simulink model "FOC_SVPWM_Implementation"  (R2025a)
settings: Solver=FixedStepDiscrete  StartTime=0.0  StopTime=10.0  FixedStep=0.0001  RelTol=1e-3
values from neighbouring files (symbols this model uses):
  dq_decouping_ena = 1.0    [FOV_SVPWM_Algorithm.sldd]
  dq_voltage_ratio = 0.57735026918962584    [FOV_SVPWM_Algorithm.sldd]
  duty_sat_lower = 0.0    [FOV_SVPWM_Algorithm.sldd]
  duty_sat_upper = 100.0    [FOV_SVPWM_Algorithm.sldd]
  I_s_max = 350.0    [FOV_SVPWM_Algorithm.sldd]
  KI_c = 30.0    [FOV_SVPWM_Algorithm.sldd]
  Kp_c = 1.1    [FOV_SVPWM_Algorithm.sldd]
  L_d = 0.0003    [FOV_SVPWM_Algorithm.sldd]
  L_q = 0.0003    [FOV_SVPWM_Algorithm.sldd]
  p = 3.0    [FOV_SVPWM_Algorithm.sldd]
  Psi_p = 0.095    [FOV_SVPWM_Algorithm.sldd]
  svpwm_ena = 1.0    [FOV_SVPWM_Algorithm.sldd]
undefined symbols (not defined in the file or in its folder): DiscIntNeverNeededParam
libraries: simulink x4
settings Model: DataDictionary=FOV_SVPWM_Algorithm.sldd  Creator=RSINGH25  LastModifiedBy=RSINGH25
settings OptimizationCC: DefaultParameterBehavior=Inlined  EnhancedBackFolding=on  PassReuseOutputArgsThreshold=0.0  OptimizeBlockOrder=speed  DifferentSizesBufferReuse=on  OptimizationCustomize=off
settings DebuggingCC: ParameterPrecisionLossMsg=none  ParamSuppressDoubleToSinglePrecisionLossMsg=on  ParameterTunabilityLossMsg=error
settings SFSimCC: MATLABDynamicMemAlloc=off
settings RTWCC: GenCodeOnly=on  GenerateReport=on  LaunchReport=on
settings CodeAppCC: ForceParamTrailComments=on  OperatorAnnotations=on

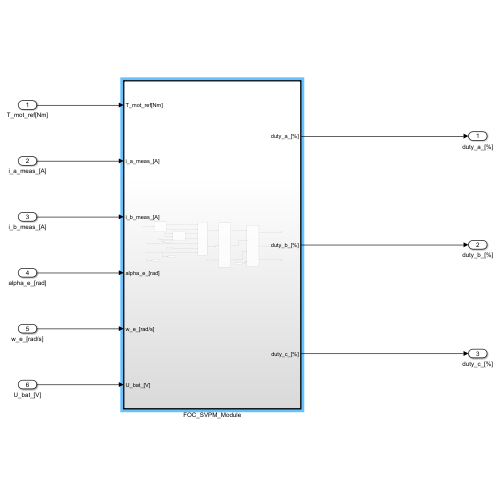
[thumbnail: Simulink's stored preview of the top-level diagram]
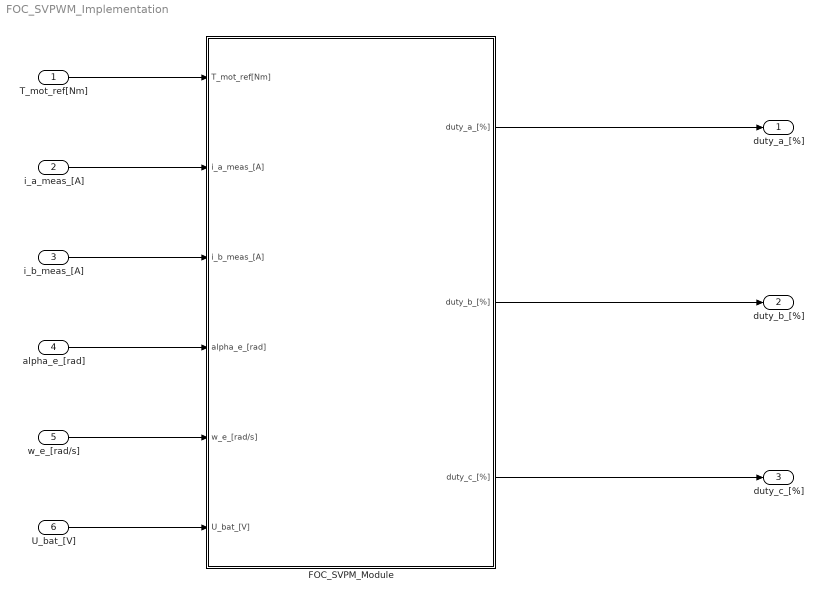
== system FOC_SVPWM_Implementation ==
  T_mot_ref[Nm] : Inport
  i_a_meas_[A] : Inport  Port=2
  i_b_meas_[A] : Inport  Port=3
  alpha_e_[rad] : Inport  Port=4
  w_e_[rad/s] : Inport  Port=5
  U_bat_[V] : Inport  Port=6
  FOC_SVPM_Module : Subsystem  TreatAsAtomicUnit=on
  duty_a_[%] : Outport
  duty_b_[%] : Outport  Port=2
  duty_c_[%] : Outport  Port=3
  wires:
  T_mot_ref[Nm]/1 -> FOC_SVPM_Module/1(T_mot_ref[Nm])
  i_a_meas_[A]/1 -> FOC_SVPM_Module/2(i_a_meas_[A])
  i_b_meas_[A]/1 -> FOC_SVPM_Module/3(i_b_meas_[A])
  alpha_e_[rad]/1 -> FOC_SVPM_Module/4(alpha_e_[rad])
  w_e_[rad/s]/1 -> FOC_SVPM_Module/5(w_e_[rad/s])
  U_bat_[V]/1 -> FOC_SVPM_Module/6(U_bat_[V])
  FOC_SVPM_Module/1(duty_a_[%]) -> duty_a_[%]/1
  FOC_SVPM_Module/2(duty_b_[%]) -> duty_b_[%]/1
  FOC_SVPM_Module/3(duty_c_[%]) -> duty_c_[%]/1

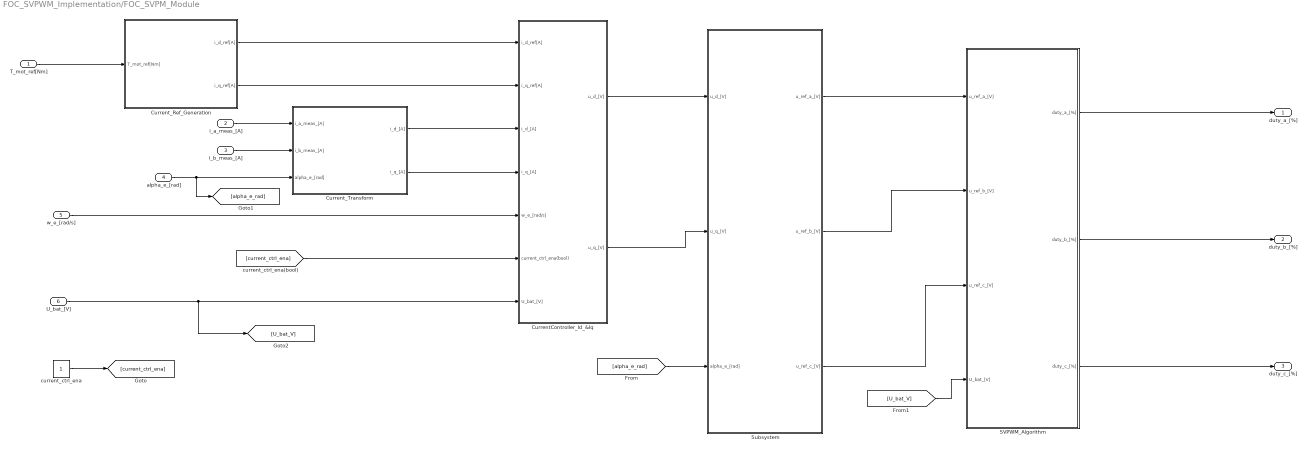
== system FOC_SVPWM_Implementation/FOC_SVPM_Module ==
  T_mot_ref[Nm] : Inport
  i_a_meas_[A] : Inport  Port=2
  i_b_meas_[A] : Inport  Port=3
  alpha_e_[rad] : Inport  Port=4
  w_e_[rad/s] : Inport  Port=5
  U_bat_[V] : Inport  Port=6
  CurrentController_Id_&Iq : Subsystem  TreatAsAtomicUnit=on
  Current_Ref_Generation : Subsystem  TreatAsAtomicUnit=on
  Current_Transform : Subsystem  TreatAsAtomicUnit=on
  SVPWM_Algorithm : Subsystem  TreatAsAtomicUnit=on
  Subsystem : Subsystem  TreatAsAtomicUnit=on
  current_ctrl_ena : Constant
  duty_a_[%] : Outport
  duty_b_[%] : Outport  Port=2
  duty_c_[%] : Outport  Port=3
  wires:
  current_ctrl_ena/1 -> [current_ctrl_ena]
  SVPWM_Algorithm/1(duty_a_[%]) -> duty_a_[%]/1
  Subsystem/2(u_ref_b_[V]) -> SVPWM_Algorithm/2(u_ref_b_[V])
  [current_ctrl_ena] -> CurrentController_Id_&Iq/6(current_ctrl_ena(bool))
  U_bat_[V]/1 -> [U_bat_V], CurrentController_Id_&Iq/7(U_bat_[V])
  Current_Transform/2(i_q_[A]) -> CurrentController_Id_&Iq/4(i_q_[A])
  Subsystem/3(u_ref_c_[V]) -> SVPWM_Algorithm/3(u_ref_c_[V])
  T_mot_ref[Nm]/1 -> Current_Ref_Generation/1(T_mot_ref[Nm])
  alpha_e_[rad]/1 -> [alpha_e_rad], Current_Transform/3(alpha_e_[rad])
  i_a_meas_[A]/1 -> Current_Transform/1(i_a_meas_[A])
  CurrentController_Id_&Iq/2(u_q_[V]) -> Subsystem/2(u_q_[V])
  CurrentController_Id_&Iq/1(u_d_[V]) -> Subsystem/1(u_d_[V])
  Current_Ref_Generation/1(i_d_ref[A]) -> CurrentController_Id_&Iq/1(i_d_ref[A])
  Current_Ref_Generation/2(i_q_ref[A]) -> CurrentController_Id_&Iq/2(i_q_ref[A])
  SVPWM_Algorithm/2(duty_b_[%]) -> duty_b_[%]/1
  Subsystem/1(u_ref_a_[V]) -> SVPWM_Algorithm/1(u_ref_a_[V])
  [U_bat_V] -> SVPWM_Algorithm/4(U_bat_[V])
  Current_Transform/1(i_d_[A]) -> CurrentController_Id_&Iq/3(i_d_[A])
  [alpha_e_rad] -> Subsystem/3(alpha_e_[rad])
  SVPWM_Algorithm/3(duty_c_[%]) -> duty_c_[%]/1
  i_b_meas_[A]/1 -> Current_Transform/2(i_b_meas_[A])
  w_e_[rad/s]/1 -> CurrentController_Id_&Iq/5(w_e_[rad/s])

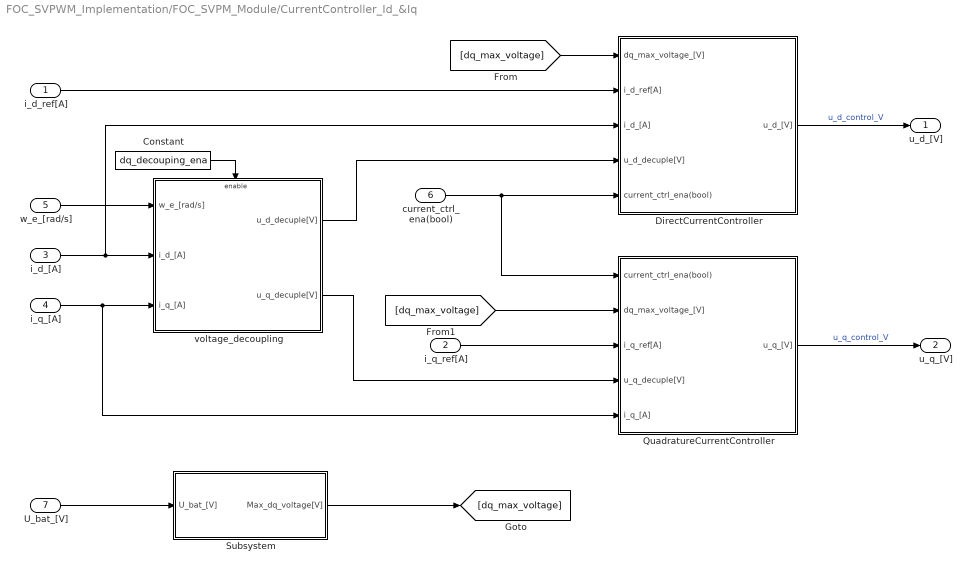
== system FOC_SVPWM_Implementation/FOC_SVPM_Module/CurrentController_Id_&Iq ==
  i_d_ref[A] : Inport
  i_q_ref[A] : Inport  Port=2
  i_d_[A] : Inport  Port=3
  i_q_[A] : Inport  Port=4
  w_e_[rad/s] : Inport  Port=5
  current_ctrl_ena(bool) : Inport  Port=6
  U_bat_[V] : Inport  Port=7
  Constant : Constant  Value=dq_decouping_ena
  DirectCurrentController : Subsystem
  QuadratureCurrentController : Subsystem
  Subsystem : Subsystem
  voltage_decoupling : Subsystem
  u_d_[V] : Outport
  u_q_[V] : Outport  Port=2
  wires:
  w_e_[rad/s]/1 -> voltage_decoupling/1(w_e_[rad/s])
  i_d_[A]/1 -> DirectCurrentController/3(i_d_[A]), voltage_decoupling/2(i_d_[A])
  i_q_[A]/1 -> QuadratureCurrentController/5(i_q_[A]), voltage_decoupling/3(i_q_[A])
  i_d_ref[A]/1 -> DirectCurrentController/2(i_d_ref[A])
  voltage_decoupling/1(u_d_decuple[V]) -> DirectCurrentController/4(u_d_decuple[V])
  current_ctrl_ena(bool)/1 -> QuadratureCurrentController/1(current_ctrl_ena(bool)), DirectCurrentController/5(current_ctrl_ena(bool))
  U_bat_[V]/1 -> Subsystem/1(U_bat_[V])
  Subsystem/1(Max_dq_voltage[V]) -> [dq_max_voltage]
  [dq_max_voltage] -> DirectCurrentController/1(dq_max_voltage_[V])
  i_q_ref[A]/1 -> QuadratureCurrentController/3(i_q_ref[A])
  voltage_decoupling/2(u_q_decuple[V]) -> QuadratureCurrentController/4(u_q_decuple[V])
  [dq_max_voltage] -> QuadratureCurrentController/2(dq_max_voltage_[V])
  DirectCurrentController/1(u_d_[V]) -> u_d_[V]/1  "u_d_control_V"
  QuadratureCurrentController/1(u_q_[V]) -> u_q_[V]/1  "u_q_control_V"
  Constant/1 -> voltage_decoupling/Enable

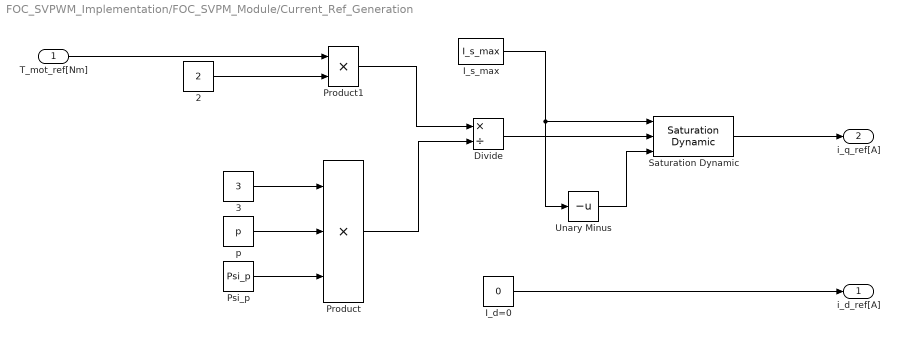
== system FOC_SVPWM_Implementation/FOC_SVPM_Module/Current_Ref_Generation ==
  T_mot_ref[Nm] : Inport
  2 : Constant  Value=2  OutDataTypeStr=single
  3 : Constant  Value=3  OutDataTypeStr=single
  Divide : Product  Inputs=*/
  I_d=0 : Constant  Value=0  OutDataTypeStr=single
  I_s_max : Constant  Value=I_s_max  OutDataTypeStr=single
  Product : Product  Inputs=3
  Product1 : Product
  Psi_p : Constant  Value=Psi_p  OutDataTypeStr=single
  Saturation Dynamic : simulink/Discontinuities/Saturation Dynamic  OutMin=[]  OutMax=[]  OutDataTypeStr=Inherit: Same as second input  OutDataType=fixdt(1, 16)  OutScaling=2^-10  DoSatur=off
  Unary Minus : UnaryMinus
  p : Constant  Value=p  OutDataTypeStr=single
  i_d_ref[A] : Outport
  i_q_ref[A] : Outport  Port=2
  wires:
  3/1 -> Product/1
  Psi_p/1 -> Product/3
  p/1 -> Product/2
  2/1 -> Product1/2
  T_mot_ref[Nm]/1 -> Product1/1
  Product1/1 -> Divide/1
  Product/1 -> Divide/2
  Saturation Dynamic/1 -> i_q_ref[A]/1
  Divide/1 -> Saturation Dynamic/2
  I_s_max/1 -> Unary Minus/1, Saturation Dynamic/1
  Unary Minus/1 -> Saturation Dynamic/3
  I_d=0/1 -> i_d_ref[A]/1

== system FOC_SVPWM_Implementation/FOC_SVPM_Module/Current_Transform ==
  i_a_meas_[A] : Inport
  i_b_meas_[A] : Inport  Port=2
  alpha_e_[rad] : Inport  Port=3
  Clark_transform : Subsystem
  Park_Transform : Subsystem
  i_d_[A] : Outport
  i_q_[A] : Outport  Port=2
  wires:
  i_a_meas_[A]/1 -> Clark_transform/1(i_a_meas_[A])
  i_b_meas_[A]/1 -> Clark_transform/2(i_b_meas_[A])
  Clark_transform/1(i_x_[A]) -> Park_Transform/1(i_x_[A])  "i_x_meas_A"
  Clark_transform/2(i_y_[A]) -> Park_Transform/2(i_y_[A])  "i_y_meas_A"
  alpha_e_[rad]/1 -> Park_Transform/3(alpha_e_[rad])
  Park_Transform/2(i_q_[A]) -> i_q_[A]/1  "i_q_meas_A"
  Park_Transform/1(i_d_[A]) -> i_d_[A]/1  "i_d_meas_A"

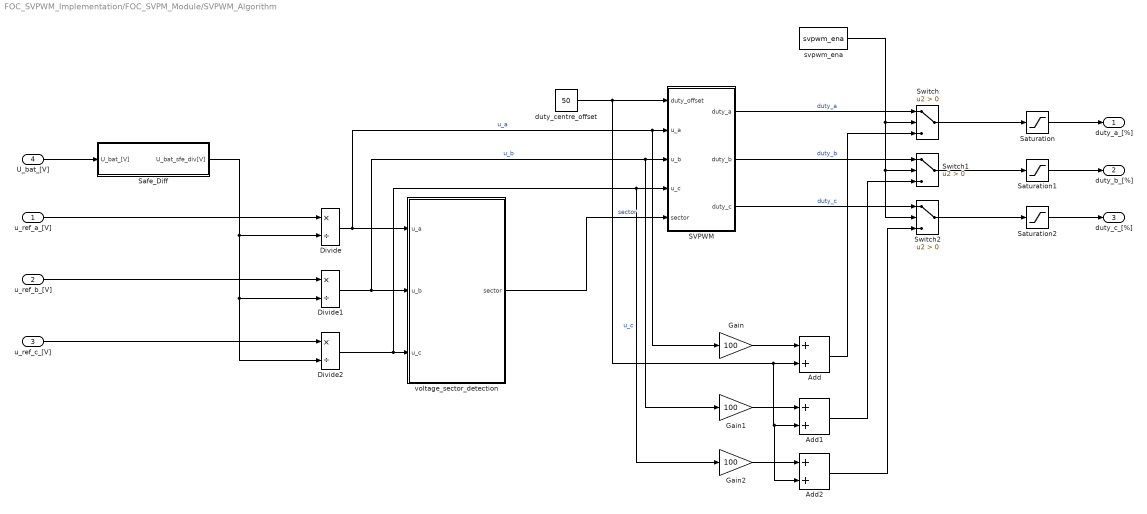
== system FOC_SVPWM_Implementation/FOC_SVPM_Module/SVPWM_Algorithm ==
  u_ref_a_[V] : Inport
  u_ref_b_[V] : Inport  Port=2
  u_ref_c_[V] : Inport  Port=3
  U_bat_[V] : Inport  Port=4
  Add : Sum
  Add1 : Sum
  Add2 : Sum
  Divide : Product  Inputs=*/
  Divide1 : Product  Inputs=*/
  Divide2 : Product  Inputs=*/
  Gain : Gain  Gain=100
  Gain1 : Gain  Gain=100
  Gain2 : Gain  Gain=100
  SVPWM : Stateflow chart  TreatAsAtomicUnit=on
  Safe_Diff : Subsystem
  Saturation : Saturate  UpperLimit=duty_sat_upper  LowerLimit=duty_sat_lower
  Saturation1 : Saturate  UpperLimit=duty_sat_upper  LowerLimit=duty_sat_lower
  Saturation2 : Saturate  UpperLimit=duty_sat_upper  LowerLimit=duty_sat_lower
  Switch : Switch  Criteria=u2 > Threshold  SaturateOnIntegerOverflow=off  InputSameDT=off
  Switch1 : Switch  Criteria=u2 > Threshold  SaturateOnIntegerOverflow=off  InputSameDT=off
  Switch2 : Switch  Criteria=u2 > Threshold  SaturateOnIntegerOverflow=off  InputSameDT=off
  duty_centre_offset : Constant  Value=50  OutDataTypeStr=single
  svpwm_ena : Constant  Value=svpwm_ena  OutDataTypeStr=single
  voltage_sector_detection : Stateflow chart  TreatAsAtomicUnit=on
  duty_a_[%] : Outport
  duty_b_[%] : Outport  Port=2
  duty_c_[%] : Outport  Port=3
  wires:
  U_bat_[V]/1 -> Safe_Diff/1(U_bat_[V])
  u_ref_a_[V]/1 -> Divide/1
  Safe_Diff/1(U_bat_sfe_div[V]) -> Divide2/2, Divide1/2, Divide/2
  u_ref_b_[V]/1 -> Divide1/1
  u_ref_c_[V]/1 -> Divide2/1
  Divide/1 -> voltage_sector_detection/1(u_a), Gain/1, SVPWM/2(u_a)  "u_a"
  Divide1/1 -> voltage_sector_detection/2(u_b), Gain1/1, SVPWM/3(u_b)  "u_b"
  Divide2/1 -> Gain2/1, SVPWM/4(u_c), voltage_sector_detection/3(u_c)  "u_c"
  voltage_sector_detection/1(sector) -> SVPWM/5(sector)  "sector"
  duty_centre_offset/1 -> Add2/2, Add1/2, Add/2, SVPWM/1(duty_offset)
  Gain/1 -> Add/1
  Gain1/1 -> Add1/1
  Gain2/1 -> Add2/1
  SVPWM/1(duty_a) -> Switch/1  "duty_a"
  SVPWM/2(duty_b) -> Switch1/1  "duty_b"
  SVPWM/3(duty_c) -> Switch2/1  "duty_c"
  Add/1 -> Switch/3
  Add1/1 -> Switch1/3
  Add2/1 -> Switch2/3
  svpwm_ena/1 -> Switch1/2, Switch2/2, Switch/2
  Switch/1 -> Saturation/1
  Switch1/1 -> Saturation1/1
  Switch2/1 -> Saturation2/1
  Saturation/1 -> duty_a_[%]/1
  Saturation1/1 -> duty_b_[%]/1
  Saturation2/1 -> duty_c_[%]/1

== system FOC_SVPWM_Implementation/FOC_SVPM_Module/Subsystem ==
  u_d_[V] : Inport
  u_q_[V] : Inport  Port=2
  alpha_e_[rad] : Inport  Port=3
  Inverse_Clark_System : Subsystem
  Inverse_Park_transform : Subsystem
  u_ref_a_[V] : Outport
  u_ref_b_[V] : Outport  Port=2
  u_ref_c_[V] : Outport  Port=3
  wires:
  u_d_[V]/1 -> Inverse_Park_transform/1(u_d_[V])
  u_q_[V]/1 -> Inverse_Park_transform/2(u_q_[V])
  alpha_e_[rad]/1 -> Inverse_Park_transform/3(alpha_e_[rad])
  Inverse_Park_transform/1(u_x_[V]) -> Inverse_Clark_System/1(u_x_[V])  "u_x_V"
  Inverse_Park_transform/2(u_y_[V]) -> Inverse_Clark_System/2(u_y_[V])  "u_y_V"
  Inverse_Clark_System/1(u_ref_a[V]) -> u_ref_a_[V]/1  "u_ref_a_V"
  Inverse_Clark_System/2(u_ref_b[V]) -> u_ref_b_[V]/1  "u_ref_b_V"
  Inverse_Clark_System/3(u_ref_c[V]) -> u_ref_c_[V]/1  "u_ref_c_V"

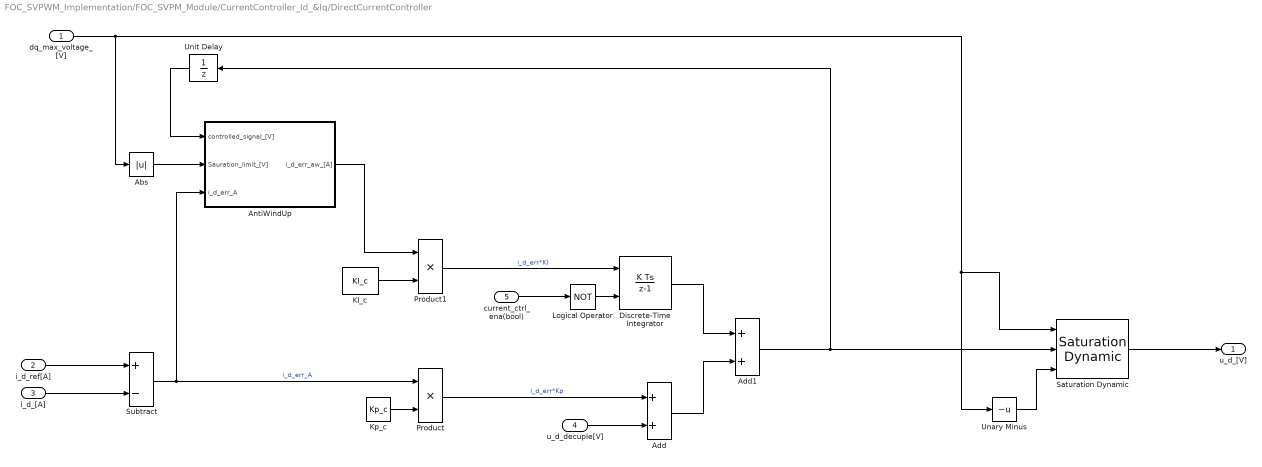
== system FOC_SVPWM_Implementation/FOC_SVPM_Module/CurrentController_Id_&Iq/DirectCurrentController ==
  dq_max_voltage_[V] : Inport
  i_d_ref[A] : Inport  Port=2
  i_d_[A] : Inport  Port=3
  u_d_decuple[V] : Inport  Port=4
  current_ctrl_ena(bool) : Inport  Port=5
  Abs : Abs  SaturateOnIntegerOverflow=off
  Add : Sum
  Add1 : Sum
  AntiWindUp : Subsystem
  Discrete-Time Integrator : DiscreteIntegrator  ExternalReset=level  SampleTime=-1  ICPrevOutput=DiscIntNeverNeededParam  ICPrevScaledInput=DiscIntNeverNeededParam
  KI_c : Constant  Value=KI_c
  Kp_c : Constant  Value=Kp_c
  Logical Operator : Logic  Operator=NOT  AllPortsSameDT=off  OutDataTypeStr=boolean
  Product : Product
  Product1 : Product
  Saturation Dynamic : simulink/Discontinuities/Saturation Dynamic  OutMin=[]  OutMax=[]  OutDataTypeStr=Inherit: Same as second input  OutDataType=fixdt(1, 16)  OutScaling=2^-10  DoSatur=off
  Subtract : Sum  Inputs=+-
  Unary Minus : UnaryMinus
  Unit Delay : UnitDelay  SampleTime=-1  HasFrameUpgradeWarning=on
  u_d_[V] : Outport
  wires:
  i_d_ref[A]/1 -> Subtract/1
  i_d_[A]/1 -> Subtract/2
  Subtract/1 -> AntiWindUp/3(i_d_err_A), Product/1  "i_d_err_A"
  Kp_c/1 -> Product/2
  Product/1 -> Add/1  "i_d_err*Kp"
  u_d_decuple[V]/1 -> Add/2
  Product1/1 -> Discrete-Time Integrator/1  "i_d_err*KI"
  current_ctrl_ena(bool)/1 -> Logical Operator/1
  KI_c/1 -> Product1/2
  Logical Operator/1 -> Discrete-Time Integrator/2
  Discrete-Time Integrator/1 -> Add1/1
  Add/1 -> Add1/2
  Add1/1 -> Unit Delay/1, Saturation Dynamic/2
  dq_max_voltage_[V]/1 -> Abs/1, Unary Minus/1, Saturation Dynamic/1
  Unary Minus/1 -> Saturation Dynamic/3
  Saturation Dynamic/1 -> u_d_[V]/1
  Unit Delay/1 -> AntiWindUp/1(controlled_signal_[V])
  Abs/1 -> AntiWindUp/2(Sauration_limit_[V])
  AntiWindUp/1(i_d_err_aw_[A]) -> Product1/1

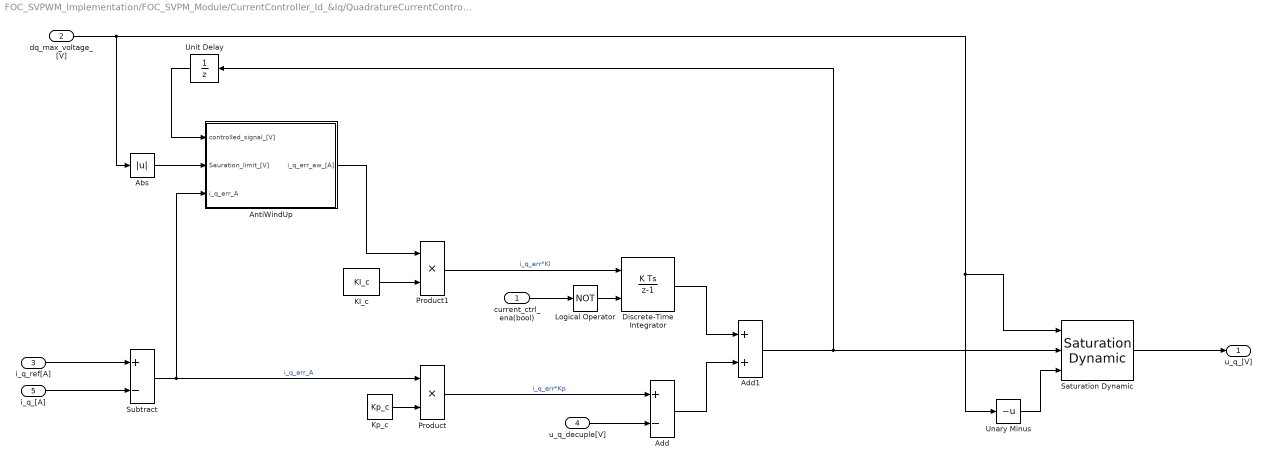
== system FOC_SVPWM_Implementation/FOC_SVPM_Module/CurrentController_Id_&Iq/QuadratureCurrentController ==
  current_ctrl_ena(bool) : Inport
  dq_max_voltage_[V] : Inport  Port=2
  i_q_ref[A] : Inport  Port=3
  u_q_decuple[V] : Inport  Port=4
  i_q_[A] : Inport  Port=5
  Abs : Abs  SaturateOnIntegerOverflow=off
  Add : Sum  Inputs=+-
  Add1 : Sum
  AntiWindUp : Subsystem
  Discrete-Time Integrator : DiscreteIntegrator  ExternalReset=level  SampleTime=-1  ICPrevOutput=DiscIntNeverNeededParam  ICPrevScaledInput=DiscIntNeverNeededParam
  KI_c : Constant  Value=KI_c
  Kp_c : Constant  Value=Kp_c
  Logical Operator : Logic  Operator=NOT  AllPortsSameDT=off  OutDataTypeStr=boolean
  Product : Product
  Product1 : Product
  Saturation Dynamic : simulink/Discontinuities/Saturation Dynamic  OutMin=[]  OutMax=[]  OutDataTypeStr=Inherit: Same as second input  OutDataType=fixdt(1, 16)  OutScaling=2^-10  DoSatur=off
  Subtract : Sum  Inputs=+-
  Unary Minus : UnaryMinus
  Unit Delay : UnitDelay  SampleTime=-1  HasFrameUpgradeWarning=on
  u_q_[V] : Outport
  wires:
  AntiWindUp/1(i_q_err_aw_[A]) -> Product1/1
  Abs/1 -> AntiWindUp/2(Sauration_limit_[V])
  Unit Delay/1 -> AntiWindUp/1(controlled_signal_[V])
  Saturation Dynamic/1 -> u_q_[V]/1
  Unary Minus/1 -> Saturation Dynamic/3
  dq_max_voltage_[V]/1 -> Saturation Dynamic/1, Unary Minus/1, Abs/1
  Add1/1 -> Saturation Dynamic/2, Unit Delay/1
  Add/1 -> Add1/2
  Discrete-Time Integrator/1 -> Add1/1
  Logical Operator/1 -> Discrete-Time Integrator/2
  KI_c/1 -> Product1/2
  current_ctrl_ena(bool)/1 -> Logical Operator/1
  Product1/1 -> Discrete-Time Integrator/1  "i_q_err*KI"
  u_q_decuple[V]/1 -> Add/2
  Product/1 -> Add/1  "i_q_err*Kp"
  Kp_c/1 -> Product/2
  Subtract/1 -> Product/1, AntiWindUp/3(i_q_err_A)  "i_q_err_A"
  i_q_[A]/1 -> Subtract/2
  i_q_ref[A]/1 -> Subtract/1

== system FOC_SVPWM_Implementation/FOC_SVPM_Module/CurrentController_Id_&Iq/Subsystem ==
  U_bat_[V] : Inport
  1/sqrt(3) : Constant  Value=dq_voltage_ratio
  Product : Product
  Max_dq_voltage[V] : Outport
  wires:
  U_bat_[V]/1 -> Product/1
  1/sqrt(3)/1 -> Product/2
  Product/1 -> Max_dq_voltage[V]/1  "dq_max_voltage_V"

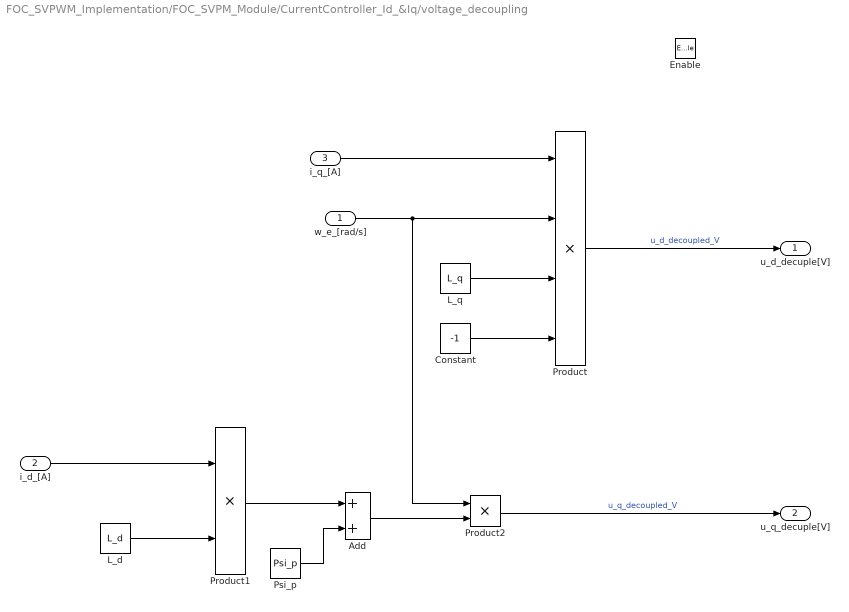
== system FOC_SVPWM_Implementation/FOC_SVPM_Module/CurrentController_Id_&Iq/voltage_decoupling ==
  w_e_[rad/s] : Inport
  i_d_[A] : Inport  Port=2
  i_q_[A] : Inport  Port=3
  Enable : EnablePort
  Add : Sum
  Constant : Constant  Value=-1  OutDataTypeStr=single
  L_d : Constant  Value=L_d
  L_q : Constant  Value=L_q
  Product : Product  Inputs=4
  Product1 : Product
  Product2 : Product
  Psi_p : Constant  Value=Psi_p
  u_d_decuple[V] : Outport
  u_q_decuple[V] : Outport  Port=2
  wires:
  i_q_[A]/1 -> Product/1
  w_e_[rad/s]/1 -> Product2/1, Product/2
  L_q/1 -> Product/3
  Constant/1 -> Product/4
  Product/1 -> u_d_decuple[V]/1  "u_d_decoupled_V"
  i_d_[A]/1 -> Product1/1
  L_d/1 -> Product1/2
  Product1/1 -> Add/1
  Psi_p/1 -> Add/2
  Add/1 -> Product2/2
  Product2/1 -> u_q_decuple[V]/1  "u_q_decoupled_V"

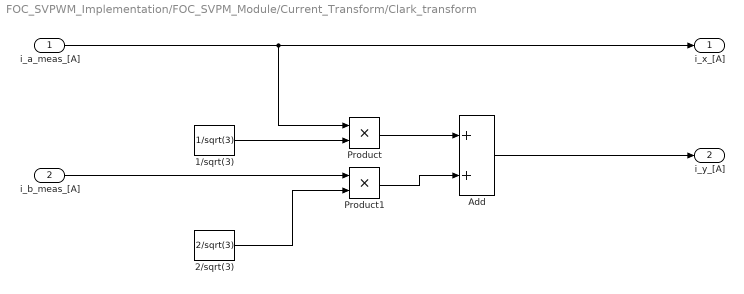
== system FOC_SVPWM_Implementation/FOC_SVPM_Module/Current_Transform/Clark_transform ==
  i_a_meas_[A] : Inport
  i_b_meas_[A] : Inport  Port=2
  1/sqrt(3) : Constant  Value=1/sqrt(3)  OutDataTypeStr=single
  2/sqrt(3) : Constant  Value=2/sqrt(3)  OutDataTypeStr=single
  Add : Sum
  Product : Product
  Product1 : Product
  i_x_[A] : Outport
  i_y_[A] : Outport  Port=2
  wires:
  i_a_meas_[A]/1 -> Product/1, i_x_[A]/1
  1/sqrt(3)/1 -> Product/2
  2/sqrt(3)/1 -> Product1/2
  i_b_meas_[A]/1 -> Product1/1
  Product/1 -> Add/1
  Product1/1 -> Add/2
  Add/1 -> i_y_[A]/1

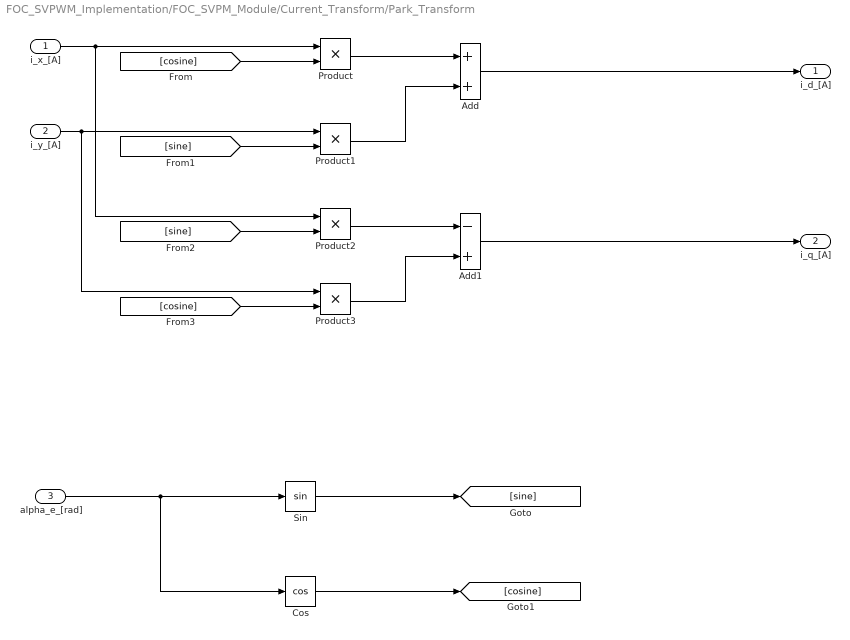
== system FOC_SVPWM_Implementation/FOC_SVPM_Module/Current_Transform/Park_Transform ==
  i_x_[A] : Inport
  i_y_[A] : Inport  Port=2
  alpha_e_[rad] : Inport  Port=3
  Add : Sum
  Add1 : Sum  Inputs=-+
  Cos : Trigonometry  Operator=cos
  Product{,1..3} (4 alike) : Product
  Sin : Trigonometry
  i_d_[A] : Outport
  i_q_[A] : Outport  Port=2
  wires:
  alpha_e_[rad]/1 -> Cos/1, Sin/1
  Sin/1 -> [sine]
  Cos/1 -> [cosine]
  i_x_[A]/1 -> Product2/1, Product/1
  [cosine] -> Product/2
  Product/1 -> Add/1
  i_y_[A]/1 -> Product3/1, Product1/1
  [sine] -> Product1/2
  Product1/1 -> Add/2
  Add/1 -> i_d_[A]/1
  Product2/1 -> Add1/1
  Product3/1 -> Add1/2
  Add1/1 -> i_q_[A]/1
  [sine] -> Product2/2
  [cosine] -> Product3/2

== system FOC_SVPWM_Implementation/FOC_SVPM_Module/SVPWM_Algorithm/Safe_Diff ==
  U_bat_[V] : Inport
  Compare To Zero : simulink/Logic and Bit Operations/Compare To Zero  relop===  OutDataTypeStr=boolean
  Constant : Constant  Value=1e-6
  Switch : Switch  Criteria=u2 > Threshold  SaturateOnIntegerOverflow=off  InputSameDT=off
  U_bat_sfe_div[V] : Outport
  wires:
  U_bat_[V]/1 -> Switch/3, Compare To Zero/1
  Compare To Zero/1 -> Switch/2
  Constant/1 -> Switch/1
  Switch/1 -> U_bat_sfe_div[V]/1

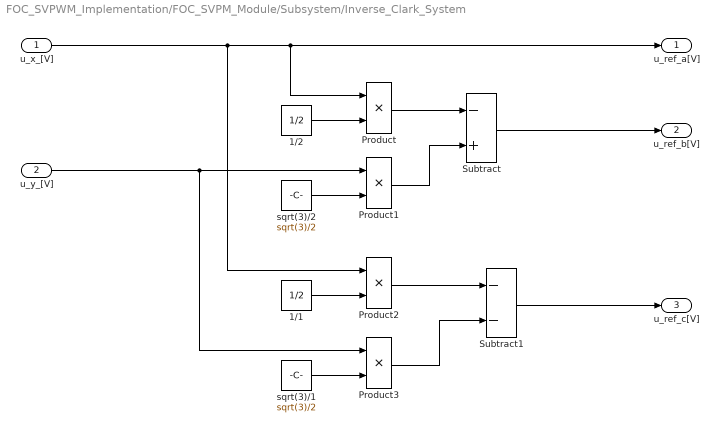
== system FOC_SVPWM_Implementation/FOC_SVPM_Module/Subsystem/Inverse_Clark_System ==
  u_x_[V] : Inport
  u_y_[V] : Inport  Port=2
  1/1 : Constant  Value=1/2  OutDataTypeStr=single
  1/2 : Constant  Value=1/2  OutDataTypeStr=single
  Product{,1..3} (4 alike) : Product
  Subtract : Sum  Inputs=-+
  Subtract1 : Sum  Inputs=--
  sqrt(3)/1 : Constant  Value=sqrt(3)/2  OutDataTypeStr=single
  sqrt(3)/2 : Constant  Value=sqrt(3)/2  OutDataTypeStr=single
  u_ref_a[V] : Outport
  u_ref_b[V] : Outport  Port=2
  u_ref_c[V] : Outport  Port=3
  wires:
  u_x_[V]/1 -> Product2/1, Product/1, u_ref_a[V]/1
  1/2/1 -> Product/2
  u_y_[V]/1 -> Product3/1, Product1/1
  sqrt(3)/2/1 -> Product1/2
  Product/1 -> Subtract/1
  Product1/1 -> Subtract/2
  Subtract/1 -> u_ref_b[V]/1
  1/1/1 -> Product2/2
  sqrt(3)/1/1 -> Product3/2
  Product2/1 -> Subtract1/1
  Product3/1 -> Subtract1/2
  Subtract1/1 -> u_ref_c[V]/1

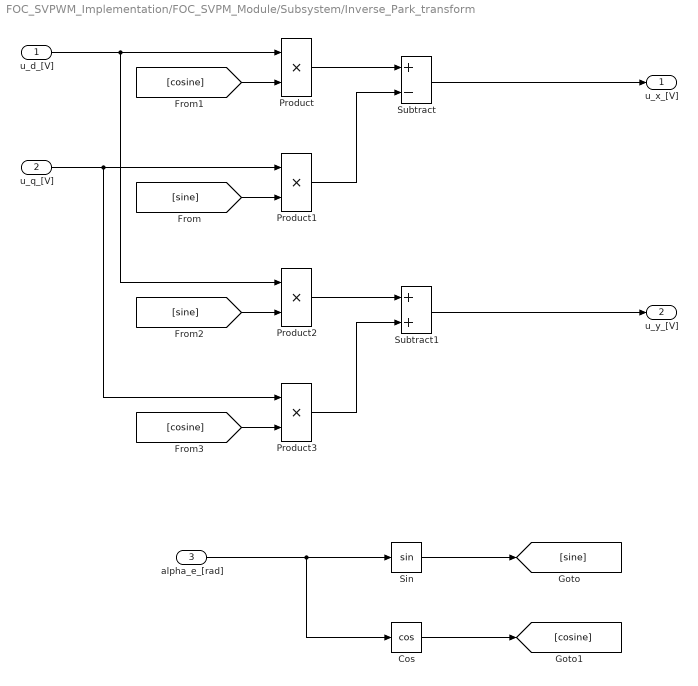
== system FOC_SVPWM_Implementation/FOC_SVPM_Module/Subsystem/Inverse_Park_transform ==
  u_d_[V] : Inport
  u_q_[V] : Inport  Port=2
  alpha_e_[rad] : Inport  Port=3
  Cos : Trigonometry  Operator=cos
  Product{,1..3} (4 alike) : Product
  Sin : Trigonometry
  Subtract : Sum  Inputs=+-
  Subtract1 : Sum
  u_x_[V] : Outport
  u_y_[V] : Outport  Port=2
  wires:
  alpha_e_[rad]/1 -> Cos/1, Sin/1
  Sin/1 -> [sine]
  Cos/1 -> [cosine]
  u_d_[V]/1 -> Product2/1, Product/1
  [cosine] -> Product/2
  u_q_[V]/1 -> Product3/1, Product1/1
  [sine] -> Product1/2
  Product/1 -> Subtract/1
  Product1/1 -> Subtract/2
  Subtract/1 -> u_x_[V]/1
  [sine] -> Product2/2
  [cosine] -> Product3/2
  Product2/1 -> Subtract1/1
  Product3/1 -> Subtract1/2
  Subtract1/1 -> u_y_[V]/1

== system FOC_SVPWM_Implementation/FOC_SVPM_Module/CurrentController_Id_&Iq/DirectCurrentController/AntiWindUp ==
  controlled_signal_[V] : Inport
  Sauration_limit_[V] : Inport  Port=2
  i_d_err_A : Inport  Port=3
  Abs : Abs  SaturateOnIntegerOverflow=off
  Product : Product
  Relational Operator : RelationalOperator  Operator=<  OutDataTypeStr=boolean  RndMeth=Simplest  InputSameDT=off
  i_d_err_aw_[A] : Outport
  wires:
  controlled_signal_[V]/1 -> Abs/1
  Abs/1 -> Relational Operator/1
  Sauration_limit_[V]/1 -> Relational Operator/2
  Relational Operator/1 -> Product/1
  i_d_err_A/1 -> Product/2
  Product/1 -> i_d_err_aw_[A]/1

== system FOC_SVPWM_Implementation/FOC_SVPM_Module/CurrentController_Id_&Iq/QuadratureCurrentController/AntiWindUp ==
  controlled_signal_[V] : Inport
  Sauration_limit_[V] : Inport  Port=2
  i_q_err_A : Inport  Port=3
  Abs : Abs  SaturateOnIntegerOverflow=off
  Product : Product
  Relational Operator : RelationalOperator  Operator=<  OutDataTypeStr=boolean  RndMeth=Simplest  InputSameDT=off
  i_q_err_aw_[A] : Outport
  wires:
  Product/1 -> i_q_err_aw_[A]/1
  i_q_err_A/1 -> Product/2
  Relational Operator/1 -> Product/1
  Sauration_limit_[V]/1 -> Relational Operator/2
  Abs/1 -> Relational Operator/1
  controlled_signal_[V]/1 -> Abs/1

== stateflow chart FOC_SVPWM_Implementation/FOC_SVPM_Module/SVPWM_Algorithm/SVPWM ==
  (default) -> (junction 10)
  (junction 10) -> (junction 12) [order 1] : [sector == 1 || sector == 4]
      | {
      | duty_a = duty_offset + duty_offset*(u_a - u_c);
      | duty_b = duty_offset + duty_offset*(2*u_b - u_a - u_c);
      | duty_c = duty_offset + duty_offset*(u_c - u_a)
      | }
  (junction 10) -> (junction 14) [order 2]
  (junction 14) -> (junction 16) [order 1] : [sector == 2 || sector == 5]
      | {
      | duty_a = duty_offset + duty_offset*(2*u_a - u_b - u_c);
      | duty_b = duty_offset + duty_offset*(u_b - u_c);
      | duty_c = duty_offset + duty_offset*(u_c - u_b)
      | }
  (junction 14) -> (junction 18) [order 2]
  (junction 18) -> (junction 20) : [sector == 3 || sector == 6]
      | {
      | duty_a = duty_offset + duty_offset*(u_a - u_b);
      | duty_b = duty_offset + duty_offset*(u_b - u_a);
      | duty_c = duty_offset + duty_offset*(2*u_c - u_a - u_b)
      | }
  data: duty_offset input; u_a input; u_b input; u_c input; sector input; duty_a output; duty_b output; duty_c output

== stateflow chart FOC_SVPWM_Implementation/FOC_SVPM_Module/SVPWM_Algorithm/voltage_sector_detection ==
  (default) -> (junction 4)
  (junction 4) -> (junction 18) [order 2]
  (junction 4) -> (junction 6) [order 1] : [u_a>=u_b]
  (junction 18) -> (junction 20)
  (junction 6) -> (junction 7) [order 1] : [u_c>=u_a]{sector = 5}
  (junction 20) -> (junction 22) [order 1] : [u_a>=u_c]{sector=2}
  (junction 6) -> (junction 10) [order 2]
  (junction 20) -> (junction 24) [order 2]
  (junction 10) -> (junction 11) [order 1] : [u_c>=u_b]{sector = 6}
  (junction 24) -> (junction 26) [order 1] : [u_b>=u_c]{sector=3}
  (junction 10) -> (junction 14) [order 2]
  (junction 24) -> (junction 28) [order 2]
  (junction 14) -> (junction 15) : {sector = 1}
  (junction 28) -> (junction 30) : {sector = 4}
  data: u_a input; u_b input; u_c input; sector output
